simulink subsystem "s_0303motor_simulator"  (R2019b)
settings: Solver=VariableStepAuto  StartTime=0.0  StopTime=10.0  RelTol=1e-3
model mask{omega_0=0, i_0=0}
  mask prompts: omega_0 "Initial Speed"; i_0 "Initial Current"
undefined symbols (not defined in the file): PARAMS
settings Model: Creator=giaco  LastModifiedBy=giaco

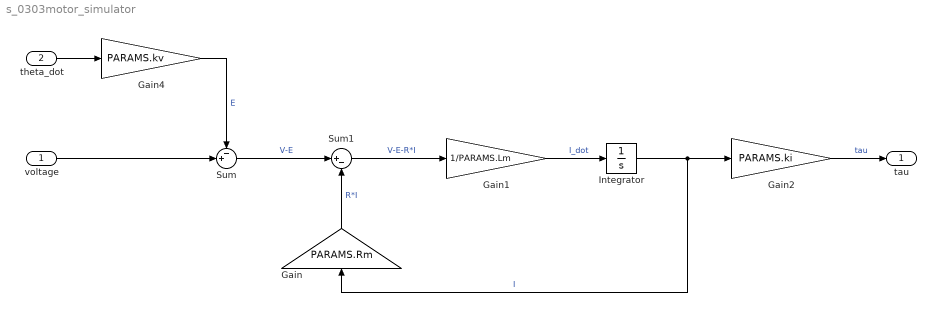
== system s_0303motor_simulator ==
  voltage : Inport
  theta_dot : Inport  Port=2
  Gain : Gain  Gain=PARAMS.Rm
  Gain1 : Gain  Gain=1/PARAMS.Lm
  Gain2 : Gain  Gain=PARAMS.ki
  Gain4 : Gain  Gain=PARAMS.kv
  Integrator : Integrator  InitialCondition=i_0
  Sum : Sum  Inputs=-+|
  Sum1 : Sum  Inputs=|+-
  tau : Outport
  wires:
  voltage/1 -> Sum/2
  Gain1/1 -> Integrator/1  "I_dot"
  Gain/1 -> Sum1/2  "R*I"
  Sum/1 -> Sum1/1  "V-E"
  Sum1/1 -> Gain1/1  "V-E-R*I"
  Integrator/1 -> Gain2/1, Gain/1  "I"
  Gain2/1 -> tau/1  "tau"
  Gain4/1 -> Sum/1  "E"
  theta_dot/1 -> Gain4/1
